simulink model "US53253_SimpleTorqueLimitingandGovernorControl"  (R2018b)
settings: Solver=ode45  StartTime=0.0  StopTime=10.0  RelTol=1e-3
undefined symbols (not defined in the file): DerivativeFilterGain_Gov, DerivativeFilterGain_Max, DerivativeFilterGain_Min, DerivativeFilterTimeConstant_Gov, DerivativeFilterTimeConstant_Max, DerivativeFilterTimeConstant_Min, DerivativeGainGovTable, DerivativeGainGovTable_X, DerivativeGainMaxTable, DerivativeGainMaxTable_X, DerivativeGainMinTable, DerivativeGainMinTable_X, DroopGovTable, DroopGovTable_X, DroopMaxTable, DroopMaxTable_X, DroopMinTable, DroopMinTable_X, FIZIT_GovSpeed, FIZIT_MaxSpeed, FIZIT_MinSpeed, FullThrottleSpeed_Gov, FullThrottleSpeed_Max, FullThrottleSpeed_Min, gov_maxspd, gov_minspd, GovTypeDefault, higpwr_C, higpwr_X, IntegralGainGovTable, IntegralGainGovTable_X, IntegralGainMinTable, IntegralGainMinTable_X, LIZIT_GovSpeed, LIZIT_MaxSpeed, LIZIT_MinSpeed, LowCoolantTempHysteresis, LowCoolantTempThreshold, lowpwr_C, lowpwr_X, LowSCRInletTempHysteresis, LowSCRInletTempThreshold, MinMaxTransitionHysteresis, nomfric_C, nomfric_X, nomfric_Y, NumberOfCylinders, ProportionalGainGovTable, ProportionalGainGovTable_X, ProportionalGainMaxTable, ProportionalGainMaxTable_X, ProportionalGainMinTable, ProportionalGainMinTable_X, SmkOp1_C, SmkOp1_X, SmkOp1_Y, ThrTqTbl_C, ThrTqTbl_X, ThrTqTbl_Y, TorqueToFuelConversionFactorInRangeTable_X ... (+8)
libraries: simulink x3, Filters x2
(part 2 of 2)

== system US53253_SimpleTorqueLimitingandGovernorControl/SimpleTorqueLimitingandGovernorController/ Torque Based Speed  Governing/governor gains/GovernorSpeedGainSelection ==
  DroopLUTableInput : Inport
  SpeedError : Inport  Port=2
  Action Port : ActionPort  ActionType=elseif
  Constant2 : Constant  Value=DerivativeFilterGain_Gov
  DerivativeGainGovTable : Lookup  InputValues=DerivativeGainGovTable_X  Table=DerivativeGainGovTable  LookUpMeth=Interpolation-Use End Values
  DroopGovTable : Lookup  InputValues=DroopGovTable_X  Table=DroopGovTable  LookUpMeth=Interpolation-Use End Values
  IntegralGainGovTable : Lookup  InputValues=IntegralGainGovTable_X  Table=IntegralGainGovTable  LookUpMeth=Interpolation-Use End Values
  ProportionalGainGovTable : Lookup  InputValues=ProportionalGainGovTable_X  Table=ProportionalGainGovTable  LookUpMeth=Interpolation-Use End Values
  Droop : Outport
  ProportionalGain : Outport  Port=2
  IntegralGain : Outport  Port=3
  DerivativeGain : Outport  Port=4
  DerivativeFilterGain : Outport  Port=5  InitialOutput=[DerivativeFilterTimeConstant_Gov]
  wires:
  DroopLUTableInput/1 -> DroopGovTable/1
  SpeedError/1 -> ProportionalGainGovTable/1, DerivativeGainGovTable/1, IntegralGainGovTable/1
  DroopGovTable/1 -> Droop/1
  ProportionalGainGovTable/1 -> ProportionalGain/1
  IntegralGainGovTable/1 -> IntegralGain/1
  DerivativeGainGovTable/1 -> DerivativeGain/1
  Constant2/1 -> DerivativeFilterGain/1

== system US53253_SimpleTorqueLimitingandGovernorControl/SimpleTorqueLimitingandGovernorController/ Torque Based Speed  Governing/governor gains/MaxSpeedGainSelection ==
  DroopLUTableInput : Inport
  SpeedError : Inport  Port=2
  Action Port : ActionPort  ActionType=else
  Constant2 : Constant  Value=DerivativeFilterGain_Max
  DerivativeGainMaxTable : Lookup  InputValues=DerivativeGainMaxTable_X  Table=DerivativeGainMaxTable  LookUpMeth=Interpolation-Use End Values
  DroopMaxTable : Lookup  InputValues=DroopMaxTable_X  Table=DroopMaxTable  LookUpMeth=Interpolation-Use End Values
  IntegralGainTable2 : Lookup  InputValues=IntegralGainGovTable_X  Table=IntegralGainGovTable  LookUpMeth=Interpolation-Use End Values
  ProportionalGainMaxTable : Lookup  InputValues=ProportionalGainMaxTable_X  Table=ProportionalGainMaxTable  LookUpMeth=Interpolation-Use End Values
  Droop : Outport
  ProportionalGain : Outport  Port=2
  IntegralGain : Outport  Port=3
  DerivativeGain : Outport  Port=4
  DerivativeFilterGain : Outport  Port=5  InitialOutput=[DerivativeFilterTimeConstant_Max]
  wires:
  DroopLUTableInput/1 -> DroopMaxTable/1
  SpeedError/1 -> ProportionalGainMaxTable/1, IntegralGainTable2/1, DerivativeGainMaxTable/1
  DroopMaxTable/1 -> Droop/1
  ProportionalGainMaxTable/1 -> ProportionalGain/1
  IntegralGainTable2/1 -> IntegralGain/1
  DerivativeGainMaxTable/1 -> DerivativeGain/1
  Constant2/1 -> DerivativeFilterGain/1

== system US53253_SimpleTorqueLimitingandGovernorControl/SimpleTorqueLimitingandGovernorController/ Torque Based Speed  Governing/governor gains/MinSpeedGainSelection ==
  DroopLUTableInput : Inport
  SpeedError : Inport  Port=2
  Action Port : ActionPort  ActionType=then
  Constant2 : Constant  Value=DerivativeFilterGain_Min
  DerivativeGainMinTable : Lookup  InputValues=DerivativeGainMinTable_X  Table=DerivativeGainMinTable  LookUpMeth=Interpolation-Use End Values
  DroopMinTable : Lookup  InputValues=DroopMinTable_X  Table=DroopMinTable  LookUpMeth=Interpolation-Use End Values
  IntegralGainMinTable : Lookup  InputValues=IntegralGainMinTable_X  Table=IntegralGainMinTable  LookUpMeth=Interpolation-Use End Values
  ProportionalGainMinTable : Lookup  InputValues=ProportionalGainMinTable_X  Table=ProportionalGainMinTable  LookUpMeth=Interpolation-Use End Values
  Droop : Outport
  ProportionalGain : Outport  Port=2
  IntegralGain : Outport  Port=3
  DerivativeGain : Outport  Port=4
  DerivativeFilterGain : Outport  Port=5  InitialOutput=[DerivativeFilterTimeConstant_Min]
  wires:
  DroopLUTableInput/1 -> DroopMinTable/1
  SpeedError/1 -> DerivativeGainMinTable/1, IntegralGainMinTable/1, ProportionalGainMinTable/1
  DroopMinTable/1 -> Droop/1
  ProportionalGainMinTable/1 -> ProportionalGain/1
  IntegralGainMinTable/1 -> IntegralGain/1
  DerivativeGainMinTable/1 -> DerivativeGain/1
  Constant2/1 -> DerivativeFilterGain/1

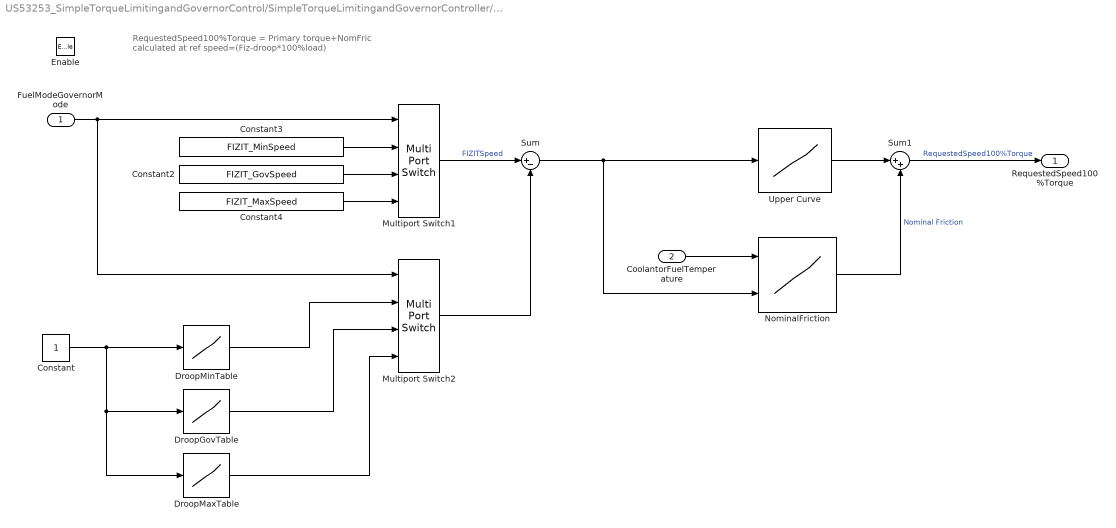
== system US53253_SimpleTorqueLimitingandGovernorControl/SimpleTorqueLimitingandGovernorController/ Torque Based Speed  Governing/governor gains/Reset Requested Speed 100% Torque with Speed Mode chagne ==
  note: RequestedSpeed100%Torque = Primary torque+NomFric
      | calculated at ref speed=(Fiz-droop*100%load)
  FuelModeGovernorMode : Inport
  CoolantorFuelTemperature : Inport  Port=2
  Enable : EnablePort
  Constant : Constant
  Constant2 : Constant  Value=FIZIT_GovSpeed
  Constant3 : Constant  Value=FIZIT_MinSpeed
  Constant4 : Constant  Value=FIZIT_MaxSpeed
  DroopGovTable : Lookup  InputValues=DroopGovTable_X  Table=DroopGovTable  LookUpMeth=Interpolation-Use End Values
  DroopMaxTable : Lookup  InputValues=DroopMaxTable_X  Table=DroopMaxTable  LookUpMeth=Interpolation-Use End Values
  DroopMinTable : Lookup  InputValues=DroopMinTable_X  Table=DroopMinTable  LookUpMeth=Interpolation-Use End Values
  Multiport Switch1 : MultiPortSwitch  DataPortOrder=Zero-based contiguous  zeroidx=on
  Multiport Switch2 : MultiPortSwitch  DataPortOrder=Zero-based contiguous  zeroidx=on
  NominalFriction : Lookup_n-D  BreakpointsForDimension1=nomfric_Y  BreakpointsForDimension2=nomfric_X  Table=nomfric_C  ExtrapMethod=Clip  UseLastTableValue=on  RndMeth=Simplest  InputSameDT=on
  Sum : Sum  Inputs=|+-
  Sum1 : Sum  Inputs=|++
  Upper Curve : Lookup  InputValues=higpwr_X  Table=higpwr_C  LookUpMeth=Interpolation-Use End Values
  RequestedSpeed100%Torque : Outport
  wires:
  Multiport Switch1/1 -> Sum/1  "FIZITSpeed"
  FuelModeGovernorMode/1 -> Multiport Switch2/1, Multiport Switch1/1
  Sum/1 -> NominalFriction/2, Upper Curve/1
  Upper Curve/1 -> Sum1/1
  Sum1/1 -> RequestedSpeed100%Torque/1  "RequestedSpeed100%Torque"
  CoolantorFuelTemperature/1 -> NominalFriction/1
  NominalFriction/1 -> Sum1/2  "Nominal Friction"
  Constant3/1 -> Multiport Switch1/2
  Constant2/1 -> Multiport Switch1/3
  Constant4/1 -> Multiport Switch1/4
  Constant/1 -> DroopMaxTable/1, DroopGovTable/1, DroopMinTable/1
  DroopMinTable/1 -> Multiport Switch2/2
  DroopGovTable/1 -> Multiport Switch2/3
  DroopMaxTable/1 -> Multiport Switch2/4
  Multiport Switch2/1 -> Sum/2

== system US53253_SimpleTorqueLimitingandGovernorControl/SimpleTorqueLimitingandGovernorController/Torque Based DesiredFuelDetermination(5ms)1/DesiredFuel/PassesDesiredFuel ==
  DesiredFuel_1 : Inport
  FuelMode_In : Inport  Port=2
  Action Port : ActionPort  ActionType=else
  DesiredFuel : Outport  InitialOutput=0
  FuelMode : Outport  Port=2  InitialOutput=0
  wires:
  DesiredFuel_1/1 -> DesiredFuel/1
  FuelMode_In/1 -> FuelMode/1

== system US53253_SimpleTorqueLimitingandGovernorControl/SimpleTorqueLimitingandGovernorController/Torque Based DesiredFuelDetermination(5ms)1/DesiredFuel/SelectsSmokeLimitAsDesiredFuel ==
  SmokeControlFuelLimit : Inport  Tag=SmokeControlFuelLimit  PortDimensions=[-1]
  FuelMode_IN : Inport  Tag=SmokeControlFuelLimit  Port=2  PortDimensions=[-1]
  Action Port : ActionPort  ActionType=then
  DesiredFuel : Outport  InitialOutput=0
  FuelMode : Outport  Port=2  InitialOutput=0
  wires:
  SmokeControlFuelLimit/1 -> DesiredFuel/1
  FuelMode_IN/1 -> FuelMode/1

== system US53253_SimpleTorqueLimitingandGovernorControl/SimpleTorqueLimitingandGovernorController/Torque Based DesiredFuelDetermination(5ms)1/DesiredFuel/Temperature_check ==
  SCRInletTemperature_C : Inport
  CoolantTemperature_C : Inport  Port=2
  Logical Operator3 : Logic  AllPortsSameDT=off
  Max_Calc_hysteresis : Subsystem
  Relational Operator : RelationalOperator  Operator=<  RndMeth=Nearest
  Relational Operator1 : RelationalOperator  Operator=<  RndMeth=Nearest
  Enable_chk : Outport
  wires:
  Max_Calc_hysteresis/2(CoolantTemp_Max_Val) -> Relational Operator1/2
  Max_Calc_hysteresis/1(SCRInletTemp_Max_Val) -> Relational Operator/2
  CoolantTemperature_C/1 -> Relational Operator1/1
  Relational Operator1/1 -> Logical Operator3/2
  SCRInletTemperature_C/1 -> Relational Operator/1
  Logical Operator3/1 -> Enable_chk/1, Max_Calc_hysteresis/1(Enable_chk)
  Relational Operator/1 -> Logical Operator3/1

== system US53253_SimpleTorqueLimitingandGovernorControl/SimpleTorqueLimitingandGovernorController/Torque Based DesiredFuelDetermination(5ms)1/DesiredFuel/Temperature_check/Max_Calc_hysteresis ==
  Enable_chk : Inport
  Logical Operator4 : Logic  Operator=NOT  AllPortsSameDT=off
  LowCoolantTemperatureHysteresis : Constant  Value=LowCoolantTempHysteresis
  LowCoolantTemperatureThrshold : Constant  Value=LowCoolantTempThreshold
  LowSCRInletTemperatureHysteresis : Constant  Value=LowSCRInletTempHysteresis
  LowSCRInletTemperatureThrshold : Constant  Value=LowSCRInletTempThreshold
  Subtract : Sum  Inputs=+-
  Subtract1 : Sum  Inputs=+-
  Switch : Switch  Criteria=u2 ~= 0
  Switch1 : Switch  Criteria=u2 ~= 0
  Unit Delay : UnitDelay  SampleTime=-1
  SCRInletTemp_Max_Val : Outport
  CoolantTemp_Max_Val : Outport  Port=2
  wires:
  Enable_chk/1 -> Logical Operator4/1
  Switch/1 -> SCRInletTemp_Max_Val/1
  Switch1/1 -> CoolantTemp_Max_Val/1
  Logical Operator4/1 -> Unit Delay/1
  Unit Delay/1 -> Switch/2, Switch1/2
  LowSCRInletTemperatureThrshold/1 -> Subtract/1, Switch/3
  Subtract1/1 -> Switch1/1
  LowCoolantTemperatureThrshold/1 -> Subtract1/1, Switch1/3
  Subtract/1 -> Switch/1
  LowSCRInletTemperatureHysteresis/1 -> Subtract/2
  LowCoolantTemperatureHysteresis/1 -> Subtract1/2

== stateflow chart US53253_SimpleTorqueLimitingandGovernorControl/SimpleTorqueLimitingandGovernorController/ Torque Based Speed  Governing/IntegralAntiWindUpLogic ==
  (default) -> (junction 4) : /* IntegralAntiWindUp */
      | {IntegClamp = 1;}
  (junction 4) -> (junction 3) [order 1] : [(!((GovernorIndicatedTorqueCommand > DesiredIndicatedTorque) && (GovSpeedError > 0))) && ...
      | (!(((GovernorIndicatedTorqueCommand < DesiredIndicatedTorque) ||(GovernorIndicatedTorqueCommand == 0.0f))...
      |  &&(GovSpeedError < 0)))]
  (junction 4) -> (junction 5) [order 2]
  (junction 3) -> (junction 2) : {IntegClamp = 0;}
  (junction 2) -> (junction 5)
  (junction 5) -> (junction 1)
  data: GovernorIndicatedTorqueCommand input double; IntegClamp output double; DesiredIndicatedTorque input double; GovSpeedError input double

== stateflow chart US53253_SimpleTorqueLimitingandGovernorControl/SimpleTorqueLimitingandGovernorController/ Torque Based Speed  Governing/GovernorIDSelection/MInMaxGovernorModeandSpeedReferneceArbitration ==
  (default) -> (junction 9) : /* MinMaxGovArbitration */
  (junction 9) -> (junction 11) [order 1] : [MaxGovTransitionSpeed <= MinGovTransitionSpeed ]
  (junction 11) -> (junction 48) : /* ModeRefSpeedMaxLessThanMin */
  (junction 9) -> (junction 10) [order 2]
  (junction 10) -> (junction 15) [order 1] : [CurrentEngineSpeed > MaxGovTransitionSpeed]
  (junction 15) -> (junction 12) : {MinMaxMode_RequestedEngineSpeed = MaximumReferenceSpeed;
      |  MinMaxFuelModeGovernorMode = 2;}
  (junction 10) -> (junction 17) [order 2]
  (junction 48) -> (junction 47) [order 1] : [MinimumReferenceSpeed >= RequestedEngineSpeed]
  (junction 47) -> (junction 46) : {MinMaxMode_RequestedEngineSpeed = MinimumReferenceSpeed;
      | MinMaxFuelModeGovernorMode = 0}
  (junction 48) -> (junction 49) [order 2] : {MinMaxMode_RequestedEngineSpeed = RequestedEngineSpeed ;
      | MinMaxFuelModeGovernorMode = 1}
  (junction 17) -> (junction 18) [order 1] : [CurrentEngineSpeed < MinGovTransitionSpeed]
  (junction 17) -> (junction 37) [order 2] : /* UsePreviousValues */
  (junction 18) -> (junction 36)
  (junction 46) -> (junction 49)
  (junction 49) -> (junction 59) : /* MaxSelect */
  (junction 37) -> (junction 36) [order 1] : [PrevMinMaxFuelModeGovernorMode == 0]
  (junction 37) -> (junction 13) [order 2] : {MinMaxMode_RequestedEngineSpeed = MaximumReferenceSpeed;
      |  MinMaxFuelModeGovernorMode = 2;}
  (junction 36) -> (junction 19) : {MinMaxMode_RequestedEngineSpeed = MinimumReferenceSpeed;
      |  MinMaxFuelModeGovernorMode = 0;}
  (junction 59) -> (junction 58) [order 1] : [MaximumReferenceSpeed <= MinMaxMode_RequestedEngineSpeed]
  (junction 59) -> (junction 16) [order 2]
  (junction 58) -> (junction 57) : {MinMaxMode_RequestedEngineSpeed = MaximumReferenceSpeed;
      | MinMaxFuelModeGovernorMode = 2}
  (junction 57) -> (junction 16)
  (junction 16) -> (junction 12)
  (junction 12) -> (junction 19)
  (junction 19) -> (junction 13)
  (junction 13) -> (junction 14)
  data: MaxGovTransitionSpeed input; MinGovTransitionSpeed input; RequestedEngineSpeed input; MinMaxFuelModeGovernorMode output; MinMaxMode_RequestedEngineSpeed output; MaximumReferenceSpeed input; MinimumReferenceSpeed input; CurrentEngineSpeed input; PrevMinMaxFuelModeGovernorMode input

== stateflow chart US53253_SimpleTorqueLimitingandGovernorControl/SimpleTorqueLimitingandGovernorController/SchedulerSubsytem ==
  settings: updateMethod=DISCRETE  sampleTime=0.005
  state task5ms [parallel]
    /* call the 5ms function */
    on every(1,tick):
    /* call the 5ms functions based on priority */
    send(TorqueBasedTorqueCurveLimiting_5ms);
    send(RequestedTorqueSelection_5ms);
    send(TorqueBasedSpeedGoverning_5ms);
    send(TorqueBasedDesiredFuelDetermination_5ms);
    settings: executionOrder=1
  state task10ms [parallel]
    /* call the 10ms function */
    entry: send(SmokeOpacity_10ms);
    settings: executionOrder=2
  events: TorqueBasedTorqueCurveLimiting_5ms output FUNCTION_CALL_EVENT; RequestedTorqueSelection_5ms output FUNCTION_CALL_EVENT; TorqueBasedSpeedGoverning_5ms output FUNCTION_CALL_EVENT; TorqueBasedDesiredFuelDetermination_5ms output FUNCTION_CALL_EVENT; SmokeOpacity_10ms output FUNCTION_CALL_EVENT
